simulink model "stable_agent_system"  (R2020b)
settings: Solver=VariableStepAuto  StartTime=0.0  StopTime=10.0  RelTol=1e-3
values from neighbouring files (symbols this model uses):
  A = A_plant - B_plant*K_plant    [alternative_model.m]    (also in alternative_model_script.m; free_response.m = sym('A', [2,2]); p1.m; stable_template.m)
  A_plant = [0 1; 880.87 0]    [alternative_model.m]    (also in alternative_model_script.m; observer_convergence.m; p1.m; stable_template.m)
  B_plant = [0; -9.9453]    [alternative_model.m]    (also in alternative_model_script.m; observer_convergence.m; p1.m; stable_template.m)
  c = 10/den    [alternative_model.m]    (also in alternative_model_script.m; p1.m = 100/den; stable_template.m; template.m)
  C = C_plant    [alternative_model.m]    (also in alternative_model_script.m; free_response.m = sym('C', [1,2]); p1.m; stable_template.m)
  C_plant = [708.27 0]    [alternative_model.m]    (also in alternative_model_script.m; observer_convergence.m; p1.m; stable_template.m)
  F = P * C' / R    [alternative_model.m]    (also in alternative_model_script.m; observer_convergence.m = P * C_plant' / R; p1.m; stable_template.m)
  K = B'/R*P    [alternative_model.m]    (also in alternative_model_script.m; free_response.m = sym('K', [2,2]); p1.m; stable_template.m)
  K_plant = acker(A_plant, B_plant, poles)    [alternative_model.m]    (also in alternative_model_script.m; p1.m; stable_template.m; template.m)
  L = -.5 * C'\P    [alternative_model.m]    (also in alternative_model_script.m; p1.m = L'; stable_template.m = L'; v2.m = L')
  output_state = 1    [v1.m]
  x0_agent = [0.1 2]    [alternative_model.m]    (also in alternative_model_script.m; p1.m = [0 0]; stable_template.m = [0 0]; template.m = [0 0])
undefined symbols (not defined in the file or in its folder): local_or_neighborhood_observer
libraries: simulink x2
settings Model: Creator=salvo  LastModifiedBy=salvo
settings ModelReferenceCC: ModelReferenceMinAlgLoopOccurrences=on

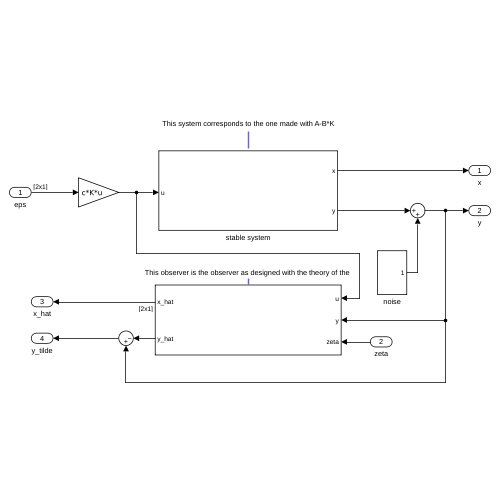
[thumbnail: Simulink's stored preview of the top-level diagram]
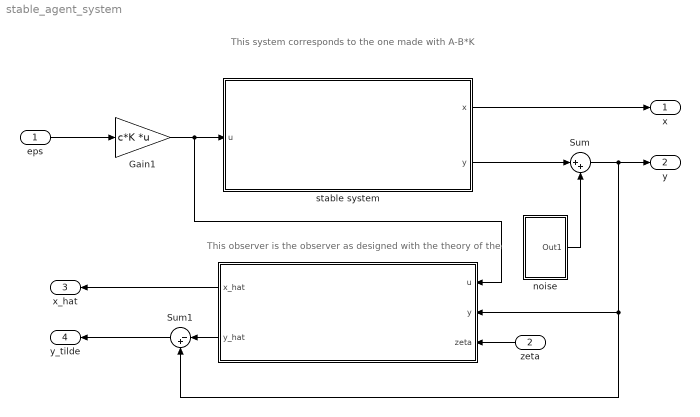
== system stable_agent_system ==
  note: This system corresponds to the one made with A-B*K
  note: This observer is the observer as designed with the theory of the
  eps : Inport  PortDimensions=[2, 1]
  zeta : Inport  Port=2
  " " : Subsystem
  Gain1 : Gain  Gain=c*K  Multiplication=Matrix(K*u)
  Sum : Sum  Inputs=|++
  Sum1 : Sum  Inputs=|-+
  noise : Subsystem
  stable system : Subsystem
  x : Outport
  y : Outport  Port=2
  x_hat : Outport  Port=3
  y_tilde : Outport  Port=4  PortDimensions=1
  wires:
  zeta/1 -> " "/3(zeta)
  Sum1/1 -> y_tilde/1
  stable system/2(y) -> Sum/1
  stable system/1(x) -> x/1
  " "/1(x_hat) -> x_hat/1
  " "/2(y_hat) -> Sum1/1
  eps/1 -> Gain1/1
  Gain1/1 -> " "/1(u), stable system/1(u)
  noise/1(Out1) -> Sum/2
  Sum/1 -> y/1, " "/2(y), Sum1/2

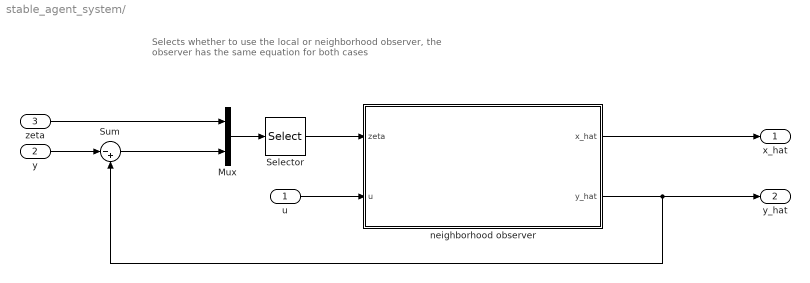
== system stable_agent_system/  ==
  note: Selects whether to use the local or neighborhood observer, the observer has the same equation for both cases
  u : Inport
  y : Inport  Port=2
  zeta : Inport  Port=3  PortDimensions=1
  Mux : Mux  Inputs=2
  Selector : Selector  InputPortWidth=2  IndexOptions=Index vector (dialog)  Indices=[local_or_neighborhood_observer]  OutputSizes=1
  Sum : Sum  Inputs=|-+
  neighborhood observer : Subsystem
  x_hat : Outport  PortDimensions=[2 1]
  y_hat : Outport  Port=2
  wires:
  u/1 -> neighborhood observer/2(u)
  neighborhood observer/1(x_hat) -> x_hat/1
  neighborhood observer/2(y_hat) -> Sum/2, y_hat/1
  y/1 -> Sum/1
  Sum/1 -> Mux/2
  Selector/1 -> neighborhood observer/1(zeta)
  Mux/1 -> Selector/1
  zeta/1 -> Mux/1

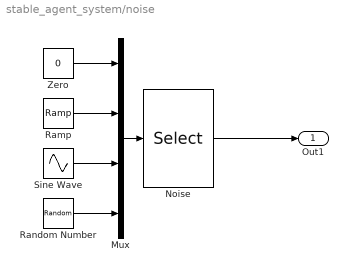
== system stable_agent_system/noise ==
  Mux : Mux
  Noise : Selector  InputPortWidth=4  IndexOptions=Index vector (dialog)  Indices=measurement_noise_type  OutputSizes=1
  Ramp : simulink/Sources/Ramp  slope=1  start=0  InitialOutput=0
  Random Number : RandomNumber  SampleTime=0.1
  Sine Wave : Sin  SampleTime=0
  Zero : Constant  Value=0  OutDataTypeStr=Inherit: Inherit via back propagation
  Out1 : Outport
  wires:
  Sine Wave/1 -> Mux/3
  Random Number/1 -> Mux/4
  Ramp/1 -> Mux/2
  Noise/1 -> Out1/1
  Zero/1 -> Mux/1
  Mux/1 -> Noise/1

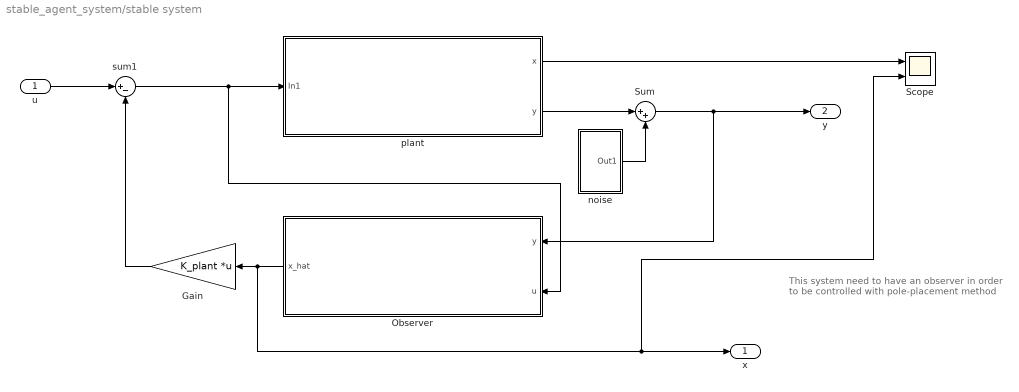
== system stable_agent_system/stable system ==
  note: This system need to have an observer in order to be controlled with pole-placement method
  u : Inport
  Gain : Gain  Gain=K_plant  Multiplication=Matrix(K*u)
  Observer : Subsystem
  Scope : Scope  NumInputPorts=2
  Sum : Sum  Inputs=|++
  noise : Subsystem
  plant : Subsystem
  sum1 : Sum  Inputs=|+-
  x : Outport
  y : Outport  Port=2
  wires:
  plant/2(y) -> Sum/1
  plant/1(x) -> Scope/1
  sum1/1 -> plant/1(In1), Observer/2(u)
  Observer/1(x_hat) -> Scope/2, x/1, Gain/1
  noise/1(Out1) -> Sum/2
  Sum/1 -> Observer/1(y), y/1
  Gain/1 -> sum1/2
  u/1 -> sum1/1

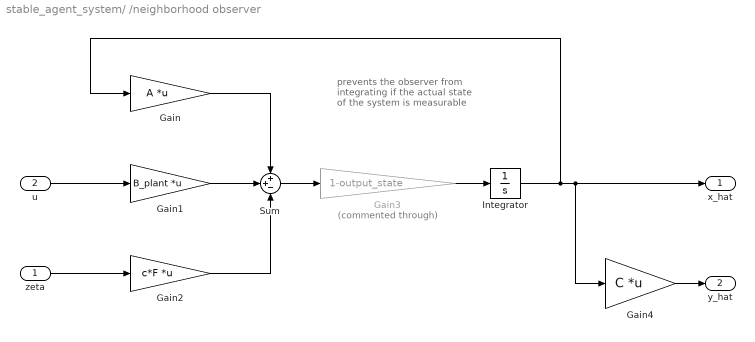
== system stable_agent_system/ /neighborhood observer ==
  note: prevents the observer from integrating if the actual state of the system is measurable
  zeta : Inport
  u : Inport  Port=2
  Gain : Gain  Gain=A  Multiplication=Matrix(K*u)
  Gain1 : Gain  Gain=B_plant  Multiplication=Matrix(K*u)
  Gain2 : Gain  Gain=c*F  Multiplication=Matrix(K*u)
  Gain3 : Gain  Commented=through  Gain=1-output_state
  Gain4 : Gain  Gain=C  Multiplication=Matrix(K*u)
  Integrator : Integrator
  Sum : Sum  Inputs=++-
  x_hat : Outport
  y_hat : Outport  Port=2
  wires:
  Integrator/1 -> Gain/1, x_hat/1, Gain4/1
  Gain/1 -> Sum/1
  Gain1/1 -> Sum/2
  u/1 -> Gain1/1
  Gain2/1 -> Sum/3
  zeta/1 -> Gain2/1
  Sum/1 -> Gain3/1
  Gain3/1 -> Integrator/1
  Gain4/1 -> y_hat/1

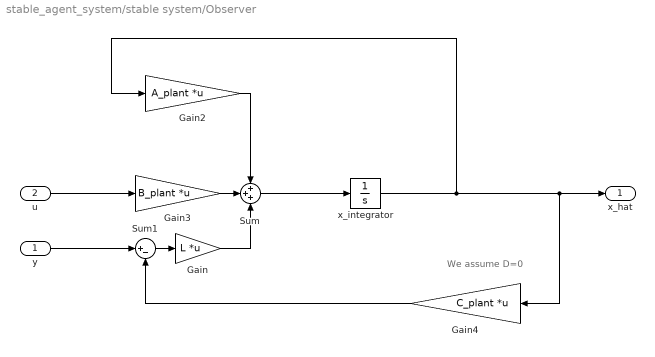
== system stable_agent_system/stable system/Observer ==
  note: We assume D=0
  y : Inport
  u : Inport  Port=2
  Gain : Gain  Gain=L  Multiplication=Matrix(K*u)
  Gain2 : Gain  Gain=A_plant  Multiplication=Matrix(K*u)
  Gain3 : Gain  Gain=B_plant  Multiplication=Matrix(K*u)
  Gain4 : Gain  Gain=C_plant  Multiplication=Matrix(K*u)
  Sum : Sum  Inputs=+++
  Sum1 : Sum  Inputs=|+-
  x_integrator : Integrator
  x_hat : Outport
  wires:
  Sum/1 -> x_integrator/1
  Gain2/1 -> Sum/1
  Gain3/1 -> Sum/2
  u/1 -> Gain3/1
  x_integrator/1 -> x_hat/1, Gain4/1, Gain2/1
  Gain4/1 -> Sum1/2
  Sum1/1 -> Gain/1
  y/1 -> Sum1/1
  Gain/1 -> Sum/3

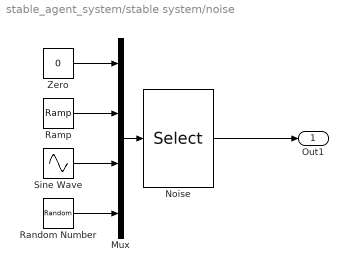
== system stable_agent_system/stable system/noise ==
  Mux : Mux
  Noise : Selector  InputPortWidth=4  IndexOptions=Index vector (dialog)  Indices=measurement_noise_type  OutputSizes=1
  Ramp : simulink/Sources/Ramp  slope=1  start=0  InitialOutput=0
  Random Number : RandomNumber  SampleTime=0.1
  Sine Wave : Sin  SampleTime=0
  Zero : Constant  Value=0  OutDataTypeStr=Inherit: Inherit via back propagation
  Out1 : Outport
  wires:
  Sine Wave/1 -> Mux/3
  Random Number/1 -> Mux/4
  Ramp/1 -> Mux/2
  Noise/1 -> Out1/1
  Zero/1 -> Mux/1
  Mux/1 -> Noise/1

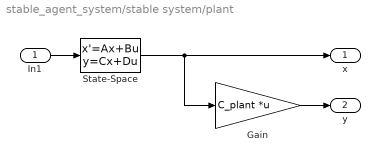
== system stable_agent_system/stable system/plant ==
  In1 : Inport
  Gain : Gain  Gain=C_plant  Multiplication=Matrix(K*u)
  State-Space : StateSpace  A=A_plant  B=B_plant  C=eye(2)  D=[0; 0]  InitialCondition=x0_agent
  x : Outport  PortDimensions=[2,1]
  y : Outport  Port=2  PortDimensions=1
  wires:
  In1/1 -> State-Space/1
  Gain/1 -> y/1
  State-Space/1 -> x/1, Gain/1
